simulink model "P702_NI_SoftECU"  (R2019a)
settings: Solver=ode1  StartTime=0.0  StopTime=Inf  FixedStep=0.001  RelTol=1e-3  EnableMultiTasking=on
PreLoadFcn:
  | run '.\VeriStand_BlockSet\NIVeriStandAddPaths.m'
undefined symbols (not defined in the file or in its folder): magnitude
libraries: simulink x83, simulink_extras x1
(part 60 of 76)

== system P702_NI_SoftECU/Output/Subsystem1/CAN_Signal/BCM ==
  in_port : Inport
  BCM_Lamp_Stat_0x3C3 : Subsystem
  Battery_Mgmt_24V_0x42E : Subsystem
  Battery_Mgmt_2_0x42C : Subsystem
  Battery_Mgmt_3_0x43C : Subsystem
  Battery_Mgmt_4_0x42B : Subsystem
  BodyInfo_3_0x3B3 : Subsystem
  Body_Info_10_0x3BA : Subsystem
  Body_Info_12_0x26E : Subsystem
  Body_Info_4_0x242 : Subsystem
  Body_Info_6_0x38D : Subsystem
  Body_Info_7_0x3B1 : Subsystem
  Body_Info_8_0x3B9 : Subsystem
  Body_Info_9_0x3A3 : Subsystem
  CMPS_FDM_Info_Status_0x3C7 : Subsystem
  CellPhonePassport_Stat_1_0x447 : Subsystem
  GGCC_Config_Mgmt_ID_1_0x40A : Subsystem
  GlobalClock_Data_0x84 : Subsystem
  Global_PATS_Control_Info2_0x42 : Subsystem
  Global_PATS_Control_Info_0x41 : Subsystem
  Locking_Systems_2_0x331 : Subsystem
  PaakRqData1_0x468 : Subsystem
  PaakRqData2_0x469 : Subsystem
  Personality_BCM2_Data_0x3EB : Subsystem
  Personality_BCM_Data_0x3E3 : Subsystem
  Power_Stat_0x456 : Subsystem
  RKE_Packet_0x3B6 : Subsystem
  TPM_Frame_0x3B7 : Subsystem
  Tire_Pressure_Data_0x3B5 : Subsystem
  Tire_Pressure_Data_DRW_0x3B8 : Subsystem
  Tire_Pressure_Stat_0x3B4 : Subsystem
  bus_selector : BusSelector  OutputSignals=Global_PATS_Control_Info_0x41,Global_PATS_Control_Info2_0x42,GlobalClock_Data_0x84,Body_Info_4_0x242,Body_Info_12_0x26E,Locking_Systems_2_0x331,Body_Info_6_0x38D,Body_Info_9_0x3A3,Body_Info_7_0x3B1,BodyInfo_3_0x3B3,Tire_Pressure_Stat_0x3B4,Tire_Pressure_Data_0x3B5,RKE_Packet_0x3B6,TPM_Frame_0x3B7,Tire_Pressure_Data_DRW_0x3B8,Body_Info_8_0x3B9,Body_Info_10_0x3BA,BCM_Lamp_Stat_0x3C3,CMPS_FDM_Info_Status_0x3C7,Personality_BCM_Data_0x3E3,Personality_BCM2_Data_0x3EB,GGCC_Config_Mgmt_ID_1_0x40A,Battery_Mgmt_4_0x42B,Battery_Mgmt_2_0x42C,Battery_Mgmt_24V_0x42E,Battery_Mgmt_3_0x43C,CellPhonePassport_Stat_1_0x447,Power_Stat_0x456,PaakRqData1_0x468,PaakRqData2_0x469
  wires:
  in_port/1 -> bus_selector/1  "Subsystem1"
  bus_selector/1 -> Global_PATS_Control_Info_0x41/1(in_port)  "<Global_PATS_Control_Info_0x41>"
  bus_selector/2 -> Global_PATS_Control_Info2_0x42/1(in_port)  "<Global_PATS_Control_Info2_0x42>"
  bus_selector/3 -> GlobalClock_Data_0x84/1(in_port)  "<GlobalClock_Data_0x84>"
  bus_selector/4 -> Body_Info_4_0x242/1(in_port)  "<Body_Info_4_0x242>"
  bus_selector/5 -> Body_Info_12_0x26E/1(in_port)  "<Body_Info_12_0x26E>"
  bus_selector/6 -> Locking_Systems_2_0x331/1(in_port)  "<Locking_Systems_2_0x331>"
  bus_selector/7 -> Body_Info_6_0x38D/1(in_port)  "<Body_Info_6_0x38D>"
  bus_selector/8 -> Body_Info_9_0x3A3/1(in_port)  "<Body_Info_9_0x3A3>"
  bus_selector/9 -> Body_Info_7_0x3B1/1(in_port)  "<Body_Info_7_0x3B1>"
  bus_selector/10 -> BodyInfo_3_0x3B3/1(in_port)  "<BodyInfo_3_0x3B3>"
  bus_selector/11 -> Tire_Pressure_Stat_0x3B4/1(in_port)  "<Tire_Pressure_Stat_0x3B4>"
  bus_selector/12 -> Tire_Pressure_Data_0x3B5/1(in_port)  "<Tire_Pressure_Data_0x3B5>"
  bus_selector/13 -> RKE_Packet_0x3B6/1(in_port)  "<RKE_Packet_0x3B6>"
  bus_selector/14 -> TPM_Frame_0x3B7/1(in_port)  "<TPM_Frame_0x3B7>"
  bus_selector/15 -> Tire_Pressure_Data_DRW_0x3B8/1(in_port)  "<Tire_Pressure_Data_DRW_0x3B8>"
  bus_selector/16 -> Body_Info_8_0x3B9/1(in_port)  "<Body_Info_8_0x3B9>"
  bus_selector/17 -> Body_Info_10_0x3BA/1(in_port)  "<Body_Info_10_0x3BA>"
  bus_selector/18 -> BCM_Lamp_Stat_0x3C3/1(in_port)  "<BCM_Lamp_Stat_0x3C3>"
  bus_selector/19 -> CMPS_FDM_Info_Status_0x3C7/1(in_port)  "<CMPS_FDM_Info_Status_0x3C7>"
  bus_selector/20 -> Personality_BCM_Data_0x3E3/1(in_port)  "<Personality_BCM_Data_0x3E3>"
  bus_selector/21 -> Personality_BCM2_Data_0x3EB/1(in_port)  "<Personality_BCM2_Data_0x3EB>"
  bus_selector/22 -> GGCC_Config_Mgmt_ID_1_0x40A/1(in_port)  "<GGCC_Config_Mgmt_ID_1_0x40A>"
  bus_selector/23 -> Battery_Mgmt_4_0x42B/1(in_port)  "<Battery_Mgmt_4_0x42B>"
  bus_selector/24 -> Battery_Mgmt_2_0x42C/1(in_port)  "<Battery_Mgmt_2_0x42C>"
  bus_selector/25 -> Battery_Mgmt_24V_0x42E/1(in_port)  "<Battery_Mgmt_24V_0x42E>"
  bus_selector/26 -> Battery_Mgmt_3_0x43C/1(in_port)  "<Battery_Mgmt_3_0x43C>"
  bus_selector/27 -> CellPhonePassport_Stat_1_0x447/1(in_port)  "<CellPhonePassport_Stat_1_0x447>"
  bus_selector/28 -> Power_Stat_0x456/1(in_port)  "<Power_Stat_0x456>"
  bus_selector/29 -> PaakRqData1_0x468/1(in_port)  "<PaakRqData1_0x468>"
  bus_selector/30 -> PaakRqData2_0x469/1(in_port)  "<PaakRqData2_0x469>"

== system P702_NI_SoftECU/Output/Subsystem1/CAN_Signal/DSMC ==
  in_port : Inport
  CMR_DSMC_AutoSar_NetwrkMgt : Subsystem
  DrvStatMonData : Subsystem
  TesterPhysicalResCMR_DSMC : Subsystem
  bus_selector : BusSelector  OutputSignals=CMR_DSMC_AutoSar_NetwrkMgt,DrvStatMonData,TesterPhysicalResCMR_DSMC
  wires:
  in_port/1 -> bus_selector/1  "Subsystem1"
  bus_selector/1 -> CMR_DSMC_AutoSar_NetwrkMgt/1(in_port)  "<CMR_DSMC_AutoSar_NetwrkMgt>"
  bus_selector/2 -> DrvStatMonData/1(in_port)  "<DrvStatMonData>"
  bus_selector/3 -> TesterPhysicalResCMR_DSMC/1(in_port)  "<TesterPhysicalResCMR_DSMC>"

== system P702_NI_SoftECU/Output/Subsystem1/CAN_Signal/ECM_DIESEL PCM PCM_HEV ==
  in_port : Inport
  EngBrakeData_0x165 : Subsystem
  EngVehicleSpThrottle2_0x202 : Subsystem
  EngVehicleSpThrottle_0x204 : Subsystem
  EngineClimateData_0x178 : Subsystem
  EngineData_6_0x156 : Subsystem
  EngineData_7_0x179 : Subsystem
  Engine_Clutch_Data_0x42F : Subsystem
  Gear_Shift_by_Wire_3 : Subsystem
  Global_PATS_TargetInfo_0x47 : Subsystem
  HEV_Powertrain_Data2 : Subsystem
  PCM_AutoSar_NetworkMgmt_0x595 : Subsystem
  PCM_Rapid_Data_Response_1_0x6A0 : Subsystem
  PowertrainData_10 : Subsystem
  PowertrainData_1_0x421 : Subsystem
  PowertrainData_2_0x42D : Subsystem
  PowertrainData_3_0x43E : Subsystem
  PowertrainData_6_0x205 : Subsystem
  PowertrainData_7_0x41F : Subsystem
  PowertrainData_9_0x44C : Subsystem
  Powertrain_Data_4_0x424 : Subsystem
  Powertrain_Data_5_0x43F : Subsystem
  Stop_Start_0x166 : Subsystem
  TesterPhysicalResPCM_0x7E8 : Subsystem
  TorqueDataEngFlags_0x200 : Subsystem
  TransGearData : Subsystem
  VehicleOperatingModes_0x167 : Subsystem
  bus_selector : BusSelector  OutputSignals=Global_PATS_TargetInfo_0x47,EngineData_6_0x156,EngBrakeData_0x165,Stop_Start_0x166,VehicleOperatingModes_0x167,EngineClimateData_0x178,EngineData_7_0x179,TorqueDataEngFlags_0x200,EngVehicleSpThrottle2_0x202,EngVehicleSpThrottle_0x204,PowertrainData_6_0x205,PowertrainData_7_0x41F,PowertrainData_1_0x421,Powertrain_Data_4_0x424,PowertrainData_2_0x42D,Engine_Clutch_Data_0x42F,PowertrainData_3_0x43E,Powertrain_Data_5_0x43F,PowertrainData_9_0x44C,PCM_AutoSar_NetworkMgmt_0x595,PCM_Rapid_Data_Response_1_0x6A0,TesterPhysicalResPCM_0x7E8,Gear_Shift_by_Wire_3,PowertrainData_10,TransGearData,HEV_Powertrain_Data2
  wires:
  in_port/1 -> bus_selector/1  "Subsystem1"
  bus_selector/1 -> Global_PATS_TargetInfo_0x47/1(in_port)  "<Global_PATS_TargetInfo_0x47>"
  bus_selector/2 -> EngineData_6_0x156/1(in_port)  "<EngineData_6_0x156>"
  bus_selector/3 -> EngBrakeData_0x165/1(in_port)  "<EngBrakeData_0x165>"
  bus_selector/4 -> Stop_Start_0x166/1(in_port)  "<Stop_Start_0x166>"
  bus_selector/5 -> VehicleOperatingModes_0x167/1(in_port)  "<VehicleOperatingModes_0x167>"
  bus_selector/6 -> EngineClimateData_0x178/1(in_port)  "<EngineClimateData_0x178>"
  bus_selector/7 -> EngineData_7_0x179/1(in_port)  "<EngineData_7_0x179>"
  bus_selector/8 -> TorqueDataEngFlags_0x200/1(in_port)  "<TorqueDataEngFlags_0x200>"
  bus_selector/9 -> EngVehicleSpThrottle2_0x202/1(in_port)  "<EngVehicleSpThrottle2_0x202>"
  bus_selector/10 -> EngVehicleSpThrottle_0x204/1(in_port)  "<EngVehicleSpThrottle_0x204>"
  bus_selector/11 -> PowertrainData_6_0x205/1(in_port)  "<PowertrainData_6_0x205>"
  bus_selector/12 -> PowertrainData_7_0x41F/1(in_port)  "<PowertrainData_7_0x41F>"
  bus_selector/13 -> PowertrainData_1_0x421/1(in_port)  "<PowertrainData_1_0x421>"
  bus_selector/14 -> Powertrain_Data_4_0x424/1(in_port)  "<Powertrain_Data_4_0x424>"
  bus_selector/15 -> PowertrainData_2_0x42D/1(in_port)  "<PowertrainData_2_0x42D>"
  bus_selector/16 -> Engine_Clutch_Data_0x42F/1(in_port)  "<Engine_Clutch_Data_0x42F>"
  bus_selector/17 -> PowertrainData_3_0x43E/1(in_port)  "<PowertrainData_3_0x43E>"
  bus_selector/18 -> Powertrain_Data_5_0x43F/1(in_port)  "<Powertrain_Data_5_0x43F>"
  bus_selector/19 -> PowertrainData_9_0x44C/1(in_port)  "<PowertrainData_9_0x44C>"
  bus_selector/20 -> PCM_AutoSar_NetworkMgmt_0x595/1(in_port)  "<PCM_AutoSar_NetworkMgmt_0x595>"
  bus_selector/21 -> PCM_Rapid_Data_Response_1_0x6A0/1(in_port)  "<PCM_Rapid_Data_Response_1_0x6A0>"
  bus_selector/22 -> TesterPhysicalResPCM_0x7E8/1(in_port)  "<TesterPhysicalResPCM_0x7E8>"
  bus_selector/23 -> Gear_Shift_by_Wire_3/1(in_port)  "<Gear_Shift_by_Wire_3>"
  bus_selector/24 -> PowertrainData_10/1(in_port)  "<PowertrainData_10>"
  bus_selector/25 -> TransGearData/1(in_port)  "<TransGearData>"
  bus_selector/26 -> HEV_Powertrain_Data2/1(in_port)  "<HEV_Powertrain_Data2>"

== system P702_NI_SoftECU/Output/Subsystem1/CAN_Signal/GWM ==
  in_port : Inport
  GSM : Subsystem
  Other_GWMTx : Subsystem
  RCM : Subsystem
  SCCM : Subsystem
  Tester/AutoSar : Subsystem
  bus_selector : BusSelector  OutputSignals=Other_GWMTx,RCM,SCCM,GSM,Tester/AutoSar
  wires:
  in_port/1 -> bus_selector/1  "Subsystem1"
  bus_selector/1 -> Other_GWMTx/1(in_port)  "<Other_GWMTx>"
  bus_selector/2 -> RCM/1(in_port)  "<RCM>"
  bus_selector/3 -> SCCM/1(in_port)  "<SCCM>"
  bus_selector/4 -> GSM/1(in_port)  "<GSM>"
  bus_selector/5 -> Tester/AutoSar/1(in_port)  "<Tester/AutoSar>"

== system P702_NI_SoftECU/Output/Subsystem1/CAN_Signal/PSCM ==
  in_port : Inport
  EPAS_INFO_0x82 : Subsystem
  Lane_Assist_Data3_FD1_0x3CC : Subsystem
  PSCM_AutoSar_NetwrkMgmt_0x5B5 : Subsystem
  SteeringPinion_Data_0x7E : Subsystem
  TesterPhysicalResPSCM_0x738 : Subsystem
  TrailerAid_Data2_0x417 : Subsystem
  bus_selector : BusSelector  OutputSignals=SteeringPinion_Data_0x7E,EPAS_INFO_0x82,Lane_Assist_Data3_FD1_0x3CC,TrailerAid_Data2_0x417,PSCM_AutoSar_NetwrkMgmt_0x5B5,TesterPhysicalResPSCM_0x738
  wires:
  in_port/1 -> bus_selector/1  "Subsystem1"
  bus_selector/1 -> SteeringPinion_Data_0x7E/1(in_port)  "<SteeringPinion_Data_0x7E>"
  bus_selector/2 -> EPAS_INFO_0x82/1(in_port)  "<EPAS_INFO_0x82>"
  bus_selector/3 -> Lane_Assist_Data3_FD1_0x3CC/1(in_port)  "<Lane_Assist_Data3_FD1_0x3CC>"
  bus_selector/4 -> TrailerAid_Data2_0x417/1(in_port)  "<TrailerAid_Data2_0x417>"
  bus_selector/5 -> PSCM_AutoSar_NetwrkMgmt_0x5B5/1(in_port)  "<PSCM_AutoSar_NetwrkMgmt_0x5B5>"
  bus_selector/6 -> TesterPhysicalResPSCM_0x738/1(in_port)  "<TesterPhysicalResPSCM_0x738>"

== system P702_NI_SoftECU/Output/Subsystem1/CAN_Signal/RealPCM ==
  in_port : Inport
  EngBrakeData : Subsystem
  EngVehicleSpThrottle2 : Subsystem
  bus_selector : BusSelector  OutputSignals=EngBrakeData,EngVehicleSpThrottle2,user_channel
  user_channel : Subsystem
  wires:
  in_port/1 -> bus_selector/1  "Subsystem1"
  bus_selector/1 -> EngBrakeData/1(in_port)  "<EngBrakeData>"
  bus_selector/2 -> EngVehicleSpThrottle2/1(in_port)  "<EngVehicleSpThrottle2>"
  bus_selector/3 -> user_channel/1(in_port)  "<user_channel>"

== system P702_NI_SoftECU/Output/Subsystem1/To_NI_HIL/DSMC ==
  in_port : Inport
  DrvStatMonData : Subsystem
  bus_selector : BusSelector  OutputSignals=DrvStatMonData
  wires:
  in_port/1 -> bus_selector/1  "Subsystem1"
  bus_selector/1 -> DrvStatMonData/1(in_port)  "<DrvStatMonData>"

== system P702_NI_SoftECU/Output/Subsystem1/To_NI_HIL/MRR ==
  in_port : Inport
  CAN_DET_AZIMUTH_01[rad] : Terminator
  CAN_DET_AZIMUTH_02[rad] : Terminator
  CAN_DET_AZIMUTH_03[rad] : Terminator
  CAN_DET_ELEVATION_01[rad] : Terminator
  CAN_DET_ELEVATION_02[rad] : Terminator
  CAN_DET_ELEVATION_03[rad] : Terminator
  CAN_DET_RANGE_01[m] : Terminator
  CAN_DET_RANGE_02[m] : Terminator
  CAN_DET_RANGE_03[m] : Terminator
  CAN_DET_RANGE_RATE_01[m/s] : Terminator
  CAN_DET_RANGE_RATE_02[m/s] : Terminator
  CAN_DET_RANGE_RATE_03[m/s] : Terminator
  bus_selector : BusSelector  OutputSignals=CAN_DET_RANGE_01[m],CAN_DET_RANGE_RATE_01[m/s],CAN_DET_AZIMUTH_01[rad],CAN_DET_ELEVATION_01[rad],CAN_DET_RANGE_02[m],CAN_DET_RANGE_RATE_02[m/s],CAN_DET_AZIMUTH_02[rad],CAN_DET_ELEVATION_02[rad],CAN_DET_RANGE_03[m],CAN_DET_RANGE_RATE_03[m/s],CAN_DET_AZIMUTH_03[rad],CAN_DET_ELEVATION_03[rad]
  wires:
  in_port/1 -> bus_selector/1  "Subsystem1"
  bus_selector/1 -> CAN_DET_RANGE_01[m]/1  "<CAN_DET_RANGE_01[m]>"
  bus_selector/2 -> CAN_DET_RANGE_RATE_01[m/s]/1  "<CAN_DET_RANGE_RATE_01[m/s]>"
  bus_selector/3 -> CAN_DET_AZIMUTH_01[rad]/1  "<CAN_DET_AZIMUTH_01[rad]>"
  bus_selector/4 -> CAN_DET_ELEVATION_01[rad]/1  "<CAN_DET_ELEVATION_01[rad]>"
  bus_selector/5 -> CAN_DET_RANGE_02[m]/1  "<CAN_DET_RANGE_02[m]>"
  bus_selector/6 -> CAN_DET_RANGE_RATE_02[m/s]/1  "<CAN_DET_RANGE_RATE_02[m/s]>"
  bus_selector/7 -> CAN_DET_AZIMUTH_02[rad]/1  "<CAN_DET_AZIMUTH_02[rad]>"
  bus_selector/8 -> CAN_DET_ELEVATION_02[rad]/1  "<CAN_DET_ELEVATION_02[rad]>"
  bus_selector/9 -> CAN_DET_RANGE_03[m]/1  "<CAN_DET_RANGE_03[m]>"
  bus_selector/10 -> CAN_DET_RANGE_RATE_03[m/s]/1  "<CAN_DET_RANGE_RATE_03[m/s]>"
  bus_selector/11 -> CAN_DET_AZIMUTH_03[rad]/1  "<CAN_DET_AZIMUTH_03[rad]>"
  bus_selector/12 -> CAN_DET_ELEVATION_03[rad]/1  "<CAN_DET_ELEVATION_03[rad]>"

== system P702_NI_SoftECU/Output/Subsystem1/To_NI_HIL/SRR_L ==
  in_port : Inport
  FL_SOD : Subsystem
  RL_SOD : Subsystem
  bus_selector : BusSelector  OutputSignals=RL_SOD,FL_SOD
  wires:
  in_port/1 -> bus_selector/1  "Subsystem1"
  bus_selector/1 -> RL_SOD/1(in_port)  "<RL_SOD>"
  bus_selector/2 -> FL_SOD/1(in_port)  "<FL_SOD>"

== system P702_NI_SoftECU/Output/Subsystem1/To_NI_HIL/SRR_R ==
  in_port : Inport
  FR_SOD : Subsystem
  RR_SOD : Subsystem
  bus_selector : BusSelector  OutputSignals=RR_SOD,FR_SOD
  wires:
  in_port/1 -> bus_selector/1  "Subsystem1"
  bus_selector/1 -> RR_SOD/1(in_port)  "<RR_SOD>"
  bus_selector/2 -> FR_SOD/1(in_port)  "<FR_SOD>"

== system P702_NI_SoftECU/Output/Subsystem1/To_NI_HIL/Soft_ABS ==
  in_port : Inport
  ABS_BrkBst_Data : Subsystem
  Accel_Data : Subsystem
  BrakeSnData_3 : Subsystem
  BrakeSnData_4 : Subsystem
  BrakeSnData_5 : Subsystem
  BrakeSysFeatures : Subsystem
  BrakeSysFeatures_2 : Subsystem
  DesiredTorqBrk : Subsystem
  ToCarSim : Subsystem
  WheelData : Subsystem
  WheelSpeed : Subsystem
  Yaw_Data : Subsystem
  bus_selector : BusSelector  OutputSignals=WheelSpeed,WheelData,Accel_Data,Yaw_Data,BrakeSnData_3,DesiredTorqBrk,BrakeSnData_4,BrakeSysFeatures,BrakeSnData_5,ToCarSim,ABS_BrkBst_Data,BrakeSysFeatures_2
  wires:
  in_port/1 -> bus_selector/1  "Subsystem1"
  bus_selector/1 -> WheelSpeed/1(in_port)  "<WheelSpeed>"
  bus_selector/2 -> WheelData/1(in_port)  "<WheelData>"
  bus_selector/3 -> Accel_Data/1(in_port)  "<Accel_Data>"
  bus_selector/4 -> Yaw_Data/1(in_port)  "<Yaw_Data>"
  bus_selector/5 -> BrakeSnData_3/1(in_port)  "<BrakeSnData_3>"
  bus_selector/6 -> DesiredTorqBrk/1(in_port)  "<DesiredTorqBrk>"
  bus_selector/7 -> BrakeSnData_4/1(in_port)  "<BrakeSnData_4>"
  bus_selector/8 -> BrakeSysFeatures/1(in_port)  "<BrakeSysFeatures>"
  bus_selector/9 -> BrakeSnData_5/1(in_port)  "<BrakeSnData_5>"
  bus_selector/10 -> ToCarSim/1(in_port)  "<ToCarSim>"
  bus_selector/11 -> ABS_BrkBst_Data/1(in_port)  "<ABS_BrkBst_Data>"
  bus_selector/12 -> BrakeSysFeatures_2/1(in_port)  "<BrakeSysFeatures_2>"

== system P702_NI_SoftECU/Output/Subsystem1/To_NI_HIL/Soft_BCM ==
  in_port : Inport
  BodyInfo_3 : Subsystem
  Cluster_Info1 : Subsystem
  GGCC_Config_Mgmt_ID : Subsystem
  Personality_BCM2_Data : Subsystem
  bus_selector : BusSelector  OutputSignals=signal1,Cluster_Info1,BodyInfo_3,GGCC_Config_Mgmt_ID,signal5,signal6,Personality_BCM2_Data
  signal1 : Terminator
  signal5 : Terminator
  signal6 : Terminator
  wires:
  in_port/1 -> bus_selector/1  "Subsystem1"
  bus_selector/1 -> signal1/1  "<signal1>"
  bus_selector/5 -> signal5/1  "<signal5>"
  bus_selector/6 -> signal6/1  "<signal6>"
  bus_selector/2 -> Cluster_Info1/1(in_port)  "<Cluster_Info1>"
  bus_selector/3 -> BodyInfo_3/1(in_port)  "<BodyInfo_3>"
  bus_selector/4 -> GGCC_Config_Mgmt_ID/1(in_port)  "<GGCC_Config_Mgmt_ID>"
  bus_selector/7 -> Personality_BCM2_Data/1(in_port)  "<Personality_BCM2_Data>"

== system P702_NI_SoftECU/Output/Subsystem1/To_NI_HIL/Soft_ECM ==
  in_port : Inport
  EngBrakeData : Subsystem
  EngVehicleSpThrottle : Subsystem
  EngVehicleSpThrottle2 : Subsystem
  bus_selector : BusSelector  OutputSignals=EngVehicleSpThrottle2,EngBrakeData,EngVehicleSpThrottle
  wires:
  in_port/1 -> bus_selector/1  "Subsystem1"
  bus_selector/1 -> EngVehicleSpThrottle2/1(in_port)  "<EngVehicleSpThrottle2>"
  bus_selector/2 -> EngBrakeData/1(in_port)  "<EngBrakeData>"
  bus_selector/3 -> EngVehicleSpThrottle/1(in_port)  "<EngVehicleSpThrottle>"

== system P702_NI_SoftECU/Output/Subsystem1/To_NI_HIL/Soft_MRR ==
  in_port : Inport
  MRR_Detection : Subsystem
  NumOfDetections : Terminator
  bus_selector : BusSelector  OutputSignals=MRR_Detection,NumOfDetections
  wires:
  in_port/1 -> bus_selector/1  "Subsystem1"
  bus_selector/2 -> NumOfDetections/1  "<NumOfDetections>"
  bus_selector/1 -> MRR_Detection/1(in_port)  "<MRR_Detection>"

== system P702_NI_SoftECU/Output/Subsystem1/To_NI_HIL/Soft_PCM ==
  in_port : Inport
  EngBrakeData : Subsystem
  EngVehicleSpThottle2 : Subsystem
  EngVehicleSpThrottle : Subsystem
  EngineClimateData : Subsystem
  EngineClutchData : Subsystem
  EngineData_7 : Subsystem
  PowertrainData_10 : Subsystem
  TorqueDataEngFlags : Subsystem
  VehicleOperatingModes : Subsystem
  bus_selector : BusSelector  OutputSignals=EngBrakeData,EngineClimateData,EngineClutchData,EngVehicleSpThrottle,EngVehicleSpThottle2,VehicleOperatingModes,EngineData_7,TorqueDataEngFlags,PowertrainData_10
  wires:
  in_port/1 -> bus_selector/1  "Subsystem1"
  bus_selector/1 -> EngBrakeData/1(in_port)  "<EngBrakeData>"
  bus_selector/2 -> EngineClimateData/1(in_port)  "<EngineClimateData>"
  bus_selector/3 -> EngineClutchData/1(in_port)  "<EngineClutchData>"
  bus_selector/4 -> EngVehicleSpThrottle/1(in_port)  "<EngVehicleSpThrottle>"
  bus_selector/5 -> EngVehicleSpThottle2/1(in_port)  "<EngVehicleSpThottle2>"
  bus_selector/6 -> VehicleOperatingModes/1(in_port)  "<VehicleOperatingModes>"
  bus_selector/7 -> EngineData_7/1(in_port)  "<EngineData_7>"
  bus_selector/8 -> TorqueDataEngFlags/1(in_port)  "<TorqueDataEngFlags>"
  bus_selector/9 -> PowertrainData_10/1(in_port)  "<PowertrainData_10>"

== system P702_NI_SoftECU/Output/Subsystem1/To_NI_HIL/Soft_PSCM ==
  in_port : Inport
  Angle_SteeringWheel : Terminator
  StePinCompAnEst_D_Qf : Terminator
  StePinRelInit_An_Sns : Terminator
  StePw_B_Rq : Terminator
  SteWhlAngCounter : Terminator
  WhlAngleCs : Terminator
  bus_selector : BusSelector  OutputSignals=Angle_SteeringWheel,SteWhlAngCounter,WhlAngleCs,StePinRelInit_An_Sns,StePw_B_Rq,StePinCompAnEst_D_Qf
  wires:
  in_port/1 -> bus_selector/1  "Subsystem1"
  bus_selector/1 -> Angle_SteeringWheel/1  "<Angle_SteeringWheel>"
  bus_selector/2 -> SteWhlAngCounter/1  "<SteWhlAngCounter>"
  bus_selector/3 -> WhlAngleCs/1  "<WhlAngleCs>"
  bus_selector/4 -> StePinRelInit_An_Sns/1  "<StePinRelInit_An_Sns>"
  bus_selector/5 -> StePw_B_Rq/1  "<StePw_B_Rq>"
  bus_selector/6 -> StePinCompAnEst_D_Qf/1  "<StePinCompAnEst_D_Qf>"

== system P702_NI_SoftECU/Output/Subsystem1/To_NI_HIL/Soft_RCM ==
  in_port : Inport
  Accel_Data : Subsystem
  RCMStatusMessage2 : Subsystem
  Yaw_Data : Subsystem
  bus_selector : BusSelector  OutputSignals=Accel_Data,Yaw_Data,RCMStatusMessage2
  wires:
  in_port/1 -> bus_selector/1  "Subsystem1"
  bus_selector/1 -> Accel_Data/1(in_port)  "<Accel_Data>"
  bus_selector/2 -> Yaw_Data/1(in_port)  "<Yaw_Data>"
  bus_selector/3 -> RCMStatusMessage2/1(in_port)  "<RCMStatusMessage2>"

== system P702_NI_SoftECU/Output/Subsystem1/To_NI_HIL/Soft_SCCM ==
  in_port : Inport
  Steering_Data : Subsystem
  Steering_Wheel_Data2 : Subsystem
  bus_selector : BusSelector  OutputSignals=Steering_Data,Steering_Wheel_Data2
  wires:
  in_port/1 -> bus_selector/1  "Subsystem1"
  bus_selector/1 -> Steering_Data/1(in_port)  "<Steering_Data>"
  bus_selector/2 -> Steering_Wheel_Data2/1(in_port)  "<Steering_Wheel_Data2>"

== system P702_NI_SoftECU/Output/Subsystem1/To_NI_HIL/Soft_TCM ==
  in_port : Inport
  TransGearData : Subsystem
  bus_selector : BusSelector  OutputSignals=TransGearData
  wires:
  in_port/1 -> bus_selector/1  "Subsystem1"
  bus_selector/1 -> TransGearData/1(in_port)  "<TransGearData>"

== system P702_NI_SoftECU/Output/Subsystem2/CAN_Signal/ABS_ESC ==
  ABS_AutoSar_NetworkMgt_0x596 : Subsystem
  ABS_BrkBst_Data_0x4B0 : Subsystem
  ABS_Rapid_Data_Response_1_0x6B0 : Subsystem
  ABS_Rapid_Data_Response_2_0x6B1 : Subsystem
  ActiveFronSteering_Req_0x88 : Subsystem
  BrakeSnData_3_0x77 : Subsystem
  BrakeSnData_4_0x7D : Subsystem
  BrakeSnData_5_0x76 : Subsystem
  BrakeSnData_6_0x414 : Subsystem
  BrakeSysFeatures_0x415 : Subsystem
  BrakeSysFeatures_2_0x416 : Subsystem
  BrakeSysFeatures_3_0x41E : Subsystem
  DesiredTorqBrk_0x213 : Subsystem
  DesiredTorqBrk_2_0x214 : Subsystem
  Global_PATS_SubTarget_0x49 : Subsystem
  SelectDriveModeData2_0x44E : Subsystem
  SelectDriveModeData_0x420 : Subsystem
  SteeringPinion_Data2_0x7F : Subsystem
  TesterPhysicalResABS_0x768 : Subsystem
  TrailerBrakeData_0x412 : Subsystem
  WheelData_0x216 : Subsystem
  WheelSpeed_0x217 : Subsystem
  bus_creator : BusCreator  Inputs=22
  out_port : Outport
  wires:
  bus_creator/1 -> out_port/1  "Subsystem2"
  Global_PATS_SubTarget_0x49/1(out_port) -> bus_creator/1  "Global_PATS_SubTarget_0x49"
  BrakeSnData_5_0x76/1(out_port) -> bus_creator/2  "BrakeSnData_5_0x76"
  BrakeSnData_3_0x77/1(out_port) -> bus_creator/3  "BrakeSnData_3_0x77"
  BrakeSnData_4_0x7D/1(out_port) -> bus_creator/4  "BrakeSnData_4_0x7D"
  SteeringPinion_Data2_0x7F/1(out_port) -> bus_creator/5  "SteeringPinion_Data2_0x7F"
  ActiveFronSteering_Req_0x88/1(out_port) -> bus_creator/6  "ActiveFronSteering_Req_0x88"
  DesiredTorqBrk_0x213/1(out_port) -> bus_creator/7  "DesiredTorqBrk_0x213"
  DesiredTorqBrk_2_0x214/1(out_port) -> bus_creator/8  "DesiredTorqBrk_2_0x214"
  WheelData_0x216/1(out_port) -> bus_creator/9  "WheelData_0x216"
  WheelSpeed_0x217/1(out_port) -> bus_creator/10  "WheelSpeed_0x217"
  TrailerBrakeData_0x412/1(out_port) -> bus_creator/11  "TrailerBrakeData_0x412"
  BrakeSnData_6_0x414/1(out_port) -> bus_creator/12  "BrakeSnData_6_0x414"
  BrakeSysFeatures_0x415/1(out_port) -> bus_creator/13  "BrakeSysFeatures_0x415"
  BrakeSysFeatures_2_0x416/1(out_port) -> bus_creator/14  "BrakeSysFeatures_2_0x416"
  BrakeSysFeatures_3_0x41E/1(out_port) -> bus_creator/15  "BrakeSysFeatures_3_0x41E"
  SelectDriveModeData_0x420/1(out_port) -> bus_creator/16  "SelectDriveModeData_0x420"
  SelectDriveModeData2_0x44E/1(out_port) -> bus_creator/17  "SelectDriveModeData2_0x44E"
  ABS_BrkBst_Data_0x4B0/1(out_port) -> bus_creator/18  "ABS_BrkBst_Data_0x4B0"
  ABS_AutoSar_NetworkMgt_0x596/1(out_port) -> bus_creator/19  "ABS_AutoSar_NetworkMgt_0x596"
  ABS_Rapid_Data_Response_1_0x6B0/1(out_port) -> bus_creator/20  "ABS_Rapid_Data_Response_1_0x6B0"
  ABS_Rapid_Data_Response_2_0x6B1/1(out_port) -> bus_creator/21  "ABS_Rapid_Data_Response_2_0x6B1"
  TesterPhysicalResABS_0x768/1(out_port) -> bus_creator/22  "TesterPhysicalResABS_0x768"

== system P702_NI_SoftECU/Output/Subsystem2/CAN_Signal/ADAS ==
  ACCDATA : Subsystem
  ACCDATA_2 : Subsystem
  bus_creator : BusCreator  Inputs=2
  out_port : Outport
  wires:
  bus_creator/1 -> out_port/1  "Subsystem2"
  ACCDATA/1(out_port) -> bus_creator/1  "ACCDATA"
  ACCDATA_2/1(out_port) -> bus_creator/2  "ACCDATA_2"

== system P702_NI_SoftECU/Output/Subsystem2/CAN_Signal/BCM ==
  BCM_Lamp_Stat_0x3C3 : Subsystem
  Battery_Mgmt_24V_0x42E : Subsystem
  Battery_Mgmt_2_0x42C : Subsystem
  Battery_Mgmt_3_0x43C : Subsystem
  Battery_Mgmt_4_0x42B : Subsystem
  BodyInfo_3_0x3B3 : Subsystem
  Body_Info_10_0x3BA : Subsystem
  Body_Info_12_0x26E : Subsystem
  Body_Info_4_0x242 : Subsystem
  Body_Info_6_0x38D : Subsystem
  Body_Info_7_0x3B1 : Subsystem
  Body_Info_8_0x3B9 : Subsystem
  Body_Info_9_0x3A3 : Subsystem
  CMPS_FDM_Info_Status_0x3C7 : Subsystem
  CellPhonePassport_Stat_1_0x447 : Subsystem
  GGCC_Config_Mgmt_ID_1_0x40A : Subsystem
  GlobalClock_Data_0x84 : Subsystem
  Global_PATS_Control_Info2_0x42 : Subsystem
  Global_PATS_Control_Info_0x41 : Subsystem
  Locking_Systems_2_0x331 : Subsystem
  PaakRqData1_0x468 : Subsystem
  PaakRqData2_0x469 : Subsystem
  Personality_BCM2_Data_0x3EB : Subsystem
  Personality_BCM_Data_0x3E3 : Subsystem
  Power_Stat_0x456 : Subsystem
  RKE_Packet_0x3B6 : Subsystem
  TPM_Frame_0x3B7 : Subsystem
  Tire_Pressure_Data_0x3B5 : Subsystem
  Tire_Pressure_Data_DRW_0x3B8 : Subsystem
  Tire_Pressure_Stat_0x3B4 : Subsystem
  bus_creator : BusCreator  Inputs=30
  out_port : Outport
  wires:
  bus_creator/1 -> out_port/1  "Subsystem2"
  Global_PATS_Control_Info_0x41/1(out_port) -> bus_creator/1  "Global_PATS_Control_Info_0x41"
  Global_PATS_Control_Info2_0x42/1(out_port) -> bus_creator/2  "Global_PATS_Control_Info2_0x42"
  GlobalClock_Data_0x84/1(out_port) -> bus_creator/3  "GlobalClock_Data_0x84"
  Body_Info_4_0x242/1(out_port) -> bus_creator/4  "Body_Info_4_0x242"
  Body_Info_12_0x26E/1(out_port) -> bus_creator/5  "Body_Info_12_0x26E"
  Locking_Systems_2_0x331/1(out_port) -> bus_creator/6  "Locking_Systems_2_0x331"
  Body_Info_6_0x38D/1(out_port) -> bus_creator/7  "Body_Info_6_0x38D"
  Body_Info_9_0x3A3/1(out_port) -> bus_creator/8  "Body_Info_9_0x3A3"
  Body_Info_7_0x3B1/1(out_port) -> bus_creator/9  "Body_Info_7_0x3B1"
  BodyInfo_3_0x3B3/1(out_port) -> bus_creator/10  "BodyInfo_3_0x3B3"
  Tire_Pressure_Stat_0x3B4/1(out_port) -> bus_creator/11  "Tire_Pressure_Stat_0x3B4"
  Tire_Pressure_Data_0x3B5/1(out_port) -> bus_creator/12  "Tire_Pressure_Data_0x3B5"
  RKE_Packet_0x3B6/1(out_port) -> bus_creator/13  "RKE_Packet_0x3B6"
  TPM_Frame_0x3B7/1(out_port) -> bus_creator/14  "TPM_Frame_0x3B7"
  Tire_Pressure_Data_DRW_0x3B8/1(out_port) -> bus_creator/15  "Tire_Pressure_Data_DRW_0x3B8"
  Body_Info_8_0x3B9/1(out_port) -> bus_creator/16  "Body_Info_8_0x3B9"
  Body_Info_10_0x3BA/1(out_port) -> bus_creator/17  "Body_Info_10_0x3BA"
  BCM_Lamp_Stat_0x3C3/1(out_port) -> bus_creator/18  "BCM_Lamp_Stat_0x3C3"
  CMPS_FDM_Info_Status_0x3C7/1(out_port) -> bus_creator/19  "CMPS_FDM_Info_Status_0x3C7"
  Personality_BCM_Data_0x3E3/1(out_port) -> bus_creator/20  "Personality_BCM_Data_0x3E3"
  Personality_BCM2_Data_0x3EB/1(out_port) -> bus_creator/21  "Personality_BCM2_Data_0x3EB"
  GGCC_Config_Mgmt_ID_1_0x40A/1(out_port) -> bus_creator/22  "GGCC_Config_Mgmt_ID_1_0x40A"
  Battery_Mgmt_4_0x42B/1(out_port) -> bus_creator/23  "Battery_Mgmt_4_0x42B"
  Battery_Mgmt_2_0x42C/1(out_port) -> bus_creator/24  "Battery_Mgmt_2_0x42C"
  Battery_Mgmt_24V_0x42E/1(out_port) -> bus_creator/25  "Battery_Mgmt_24V_0x42E"
  Battery_Mgmt_3_0x43C/1(out_port) -> bus_creator/26  "Battery_Mgmt_3_0x43C"
  CellPhonePassport_Stat_1_0x447/1(out_port) -> bus_creator/27  "CellPhonePassport_Stat_1_0x447"
  Power_Stat_0x456/1(out_port) -> bus_creator/28  "Power_Stat_0x456"
  PaakRqData1_0x468/1(out_port) -> bus_creator/29  "PaakRqData1_0x468"
  PaakRqData2_0x469/1(out_port) -> bus_creator/30  "PaakRqData2_0x469"

== system P702_NI_SoftECU/Output/Subsystem2/CAN_Signal/DSMC ==
  CMR_DSMC_AutoSar_NetwrkMgt : Subsystem
  DrvStatMonData : Subsystem
  TesterPhysicalResCMR_DSMC : Subsystem
  bus_creator : BusCreator  Inputs=3
  out_port : Outport
  wires:
  bus_creator/1 -> out_port/1  "Subsystem2"
  CMR_DSMC_AutoSar_NetwrkMgt/1(out_port) -> bus_creator/1  "CMR_DSMC_AutoSar_NetwrkMgt"
  DrvStatMonData/1(out_port) -> bus_creator/2  "DrvStatMonData"
  TesterPhysicalResCMR_DSMC/1(out_port) -> bus_creator/3  "TesterPhysicalResCMR_DSMC"

== system P702_NI_SoftECU/Output/Subsystem2/CAN_Signal/ECM_DIESEL PCM PCM_HEV ==
  EngBrakeData_0x165 : Subsystem
  EngVehicleSpThrottle2_0x202 : Subsystem
  EngVehicleSpThrottle_0x204 : Subsystem
  EngineClimateData_0x178 : Subsystem
  EngineData_6_0x156 : Subsystem
  EngineData_7_0x179 : Subsystem
  Engine_Clutch_Data_0x42F : Subsystem
  Gear_Shift_by_Wire_3 : Subsystem
  Global_PATS_TargetInfo_0x47 : Subsystem
  HEV_Powertrain_Data2 : Subsystem
  PCM_AutoSar_NetworkMgmt_0x595 : Subsystem
  PCM_Rapid_Data_Response_1_0x6A0 : Subsystem
  PowertrainData_10 : Subsystem
  PowertrainData_1_0x421 : Subsystem
  PowertrainData_2_0x42D : Subsystem
  PowertrainData_3_0x43E : Subsystem
  PowertrainData_6_0x205 : Subsystem
  PowertrainData_7_0x41F : Subsystem
  PowertrainData_9_0x44C : Subsystem
  Powertrain_Data_4_0x424 : Subsystem
  Powertrain_Data_5_0x43F : Subsystem
  Stop_Start_0x166 : Subsystem
  TesterPhysicalResPCM_0x7E8 : Subsystem
  TorqueDataEngFlags_0x200 : Subsystem
  TransGearData : Subsystem
  VehicleOperatingModes_0x167 : Subsystem
  bus_creator : BusCreator  Inputs=26
  out_port : Outport
  wires:
  bus_creator/1 -> out_port/1  "Subsystem2"
  Global_PATS_TargetInfo_0x47/1(out_port) -> bus_creator/1  "Global_PATS_TargetInfo_0x47"
  EngineData_6_0x156/1(out_port) -> bus_creator/2  "EngineData_6_0x156"
  EngBrakeData_0x165/1(out_port) -> bus_creator/3  "EngBrakeData_0x165"
  Stop_Start_0x166/1(out_port) -> bus_creator/4  "Stop_Start_0x166"
  VehicleOperatingModes_0x167/1(out_port) -> bus_creator/5  "VehicleOperatingModes_0x167"
  EngineClimateData_0x178/1(out_port) -> bus_creator/6  "EngineClimateData_0x178"
  EngineData_7_0x179/1(out_port) -> bus_creator/7  "EngineData_7_0x179"
  TorqueDataEngFlags_0x200/1(out_port) -> bus_creator/8  "TorqueDataEngFlags_0x200"
  EngVehicleSpThrottle2_0x202/1(out_port) -> bus_creator/9  "EngVehicleSpThrottle2_0x202"
  EngVehicleSpThrottle_0x204/1(out_port) -> bus_creator/10  "EngVehicleSpThrottle_0x204"
  PowertrainData_6_0x205/1(out_port) -> bus_creator/11  "PowertrainData_6_0x205"
  PowertrainData_7_0x41F/1(out_port) -> bus_creator/12  "PowertrainData_7_0x41F"
  PowertrainData_1_0x421/1(out_port) -> bus_creator/13  "PowertrainData_1_0x421"
  Powertrain_Data_4_0x424/1(out_port) -> bus_creator/14  "Powertrain_Data_4_0x424"
  PowertrainData_2_0x42D/1(out_port) -> bus_creator/15  "PowertrainData_2_0x42D"
  Engine_Clutch_Data_0x42F/1(out_port) -> bus_creator/16  "Engine_Clutch_Data_0x42F"
  PowertrainData_3_0x43E/1(out_port) -> bus_creator/17  "PowertrainData_3_0x43E"
  Powertrain_Data_5_0x43F/1(out_port) -> bus_creator/18  "Powertrain_Data_5_0x43F"
  PowertrainData_9_0x44C/1(out_port) -> bus_creator/19  "PowertrainData_9_0x44C"
  PCM_AutoSar_NetworkMgmt_0x595/1(out_port) -> bus_creator/20  "PCM_AutoSar_NetworkMgmt_0x595"
  PCM_Rapid_Data_Response_1_0x6A0/1(out_port) -> bus_creator/21  "PCM_Rapid_Data_Response_1_0x6A0"
  TesterPhysicalResPCM_0x7E8/1(out_port) -> bus_creator/22  "TesterPhysicalResPCM_0x7E8"
  Gear_Shift_by_Wire_3/1(out_port) -> bus_creator/23  "Gear_Shift_by_Wire_3"
  PowertrainData_10/1(out_port) -> bus_creator/24  "PowertrainData_10"
  TransGearData/1(out_port) -> bus_creator/25  "TransGearData"
  HEV_Powertrain_Data2/1(out_port) -> bus_creator/26  "HEV_Powertrain_Data2"

== system P702_NI_SoftECU/Output/Subsystem2/CAN_Signal/GWM ==
  in : Inport
  GSM : Subsystem
  Other_GWMTx : Subsystem
  RCM : Subsystem
  SCCM : Subsystem
  Tester/AutoSar : Subsystem
  bus_creator : BusCreator  Inputs=5
  bus_selector : BusSelector  OutputSignals=Other_GWMTx,RCM,SCCM,GSM,Tester/AutoSar
  out_port : Outport
  wires:
  bus_creator/1 -> out_port/1  "Subsystem2"
  Other_GWMTx/1(out_port) -> bus_creator/1  "Other_GWMTx"
  RCM/1(out_port) -> bus_creator/2  "RCM"
  SCCM/1(out_port) -> bus_creator/3  "SCCM"
  GSM/1(out_port) -> bus_creator/4  "GSM"
  Tester/AutoSar/1(out_port) -> bus_creator/5  "Tester//AutoSar"
  bus_selector/1 -> Other_GWMTx/1(in)  "<Other_GWMTx>"
  bus_selector/2 -> RCM/1(in)  "<RCM>"
  bus_selector/3 -> SCCM/1(in)  "<SCCM>"
  bus_selector/4 -> GSM/1(in)  "<GSM>"
  bus_selector/5 -> Tester/AutoSar/1(in)  "<Tester/AutoSar>"
  in/1 -> bus_selector/1

== system P702_NI_SoftECU/Output/Subsystem2/CAN_Signal/PSCM ==
  EPAS_INFO_0x82 : Subsystem
  Lane_Assist_Data3_FD1_0x3CC : Subsystem
  PSCM_AutoSar_NetwrkMgmt_0x5B5 : Subsystem
  SteeringPinion_Data_0x7E : Subsystem
  TesterPhysicalResPSCM_0x738 : Subsystem
  TrailerAid_Data2_0x417 : Subsystem
  bus_creator : BusCreator  Inputs=6
  out_port : Outport
  wires:
  bus_creator/1 -> out_port/1  "Subsystem2"
  SteeringPinion_Data_0x7E/1(out_port) -> bus_creator/1  "SteeringPinion_Data_0x7E"
  EPAS_INFO_0x82/1(out_port) -> bus_creator/2  "EPAS_INFO_0x82"
  Lane_Assist_Data3_FD1_0x3CC/1(out_port) -> bus_creator/3  "Lane_Assist_Data3_FD1_0x3CC"
  TrailerAid_Data2_0x417/1(out_port) -> bus_creator/4  "TrailerAid_Data2_0x417"
  PSCM_AutoSar_NetwrkMgmt_0x5B5/1(out_port) -> bus_creator/5  "PSCM_AutoSar_NetwrkMgmt_0x5B5"
  TesterPhysicalResPSCM_0x738/1(out_port) -> bus_creator/6  "TesterPhysicalResPSCM_0x738"

== system P702_NI_SoftECU/Output/Subsystem2/CAN_Signal/RealPCM ==
  EngBrakeData : Subsystem
  EngVehicleSpThrottle2 : Subsystem
  bus_creator : BusCreator  Inputs=3
  user_channel : Subsystem
  out_port : Outport
  wires:
  bus_creator/1 -> out_port/1  "Subsystem2"
  EngBrakeData/1(out_port) -> bus_creator/1  "EngBrakeData"
  EngVehicleSpThrottle2/1(out_port) -> bus_creator/2  "EngVehicleSpThrottle2"
  user_channel/1(out_port) -> bus_creator/3  "user_channel"

== system P702_NI_SoftECU/Output/Subsystem2/To_NI_HIL/DSMC ==
  DrvStatMonData : Subsystem
  bus_creator : BusCreator  Inputs=1
  out_port : Outport
  wires:
  bus_creator/1 -> out_port/1  "Subsystem2"
  DrvStatMonData/1(out_port) -> bus_creator/1  "DrvStatMonData"

== system P702_NI_SoftECU/Output/Subsystem2/To_NI_HIL/MRR ==
  CAN_DET_AZIMUTH_01[rad] : Constant  Value=0
  CAN_DET_AZIMUTH_02[rad] : Constant  Value=0
  CAN_DET_AZIMUTH_03[rad] : Constant  Value=0
  CAN_DET_ELEVATION_01[rad] : Constant  Value=0
  CAN_DET_ELEVATION_02[rad] : Constant  Value=0
  CAN_DET_ELEVATION_03[rad] : Constant  Value=0
  CAN_DET_RANGE_01[m] : Constant  Value=0
  CAN_DET_RANGE_02[m] : Constant  Value=0
  CAN_DET_RANGE_03[m] : Constant  Value=0
  CAN_DET_RANGE_RATE_01[m/s] : Constant
  CAN_DET_RANGE_RATE_02[m/s] : Constant
  CAN_DET_RANGE_RATE_03[m/s] : Constant
  bus_creator : BusCreator  Inputs=12
  out_port : Outport
  wires:
  bus_creator/1 -> out_port/1  "Subsystem2"
  CAN_DET_RANGE_01[m]/1 -> bus_creator/1  "CAN_DET_RANGE_01[m]"
  CAN_DET_RANGE_RATE_01[m/s]/1 -> bus_creator/2  "CAN_DET_RANGE_RATE_01[m//s]"
  CAN_DET_AZIMUTH_01[rad]/1 -> bus_creator/3  "CAN_DET_AZIMUTH_01[rad]"
  CAN_DET_ELEVATION_01[rad]/1 -> bus_creator/4  "CAN_DET_ELEVATION_01[rad]"
  CAN_DET_RANGE_02[m]/1 -> bus_creator/5  "CAN_DET_RANGE_02[m]"
  CAN_DET_RANGE_RATE_02[m/s]/1 -> bus_creator/6  "CAN_DET_RANGE_RATE_02[m//s]"
  CAN_DET_AZIMUTH_02[rad]/1 -> bus_creator/7  "CAN_DET_AZIMUTH_02[rad]"
  CAN_DET_ELEVATION_02[rad]/1 -> bus_creator/8  "CAN_DET_ELEVATION_02[rad]"
  CAN_DET_RANGE_03[m]/1 -> bus_creator/9  "CAN_DET_RANGE_03[m]"
  CAN_DET_RANGE_RATE_03[m/s]/1 -> bus_creator/10  "CAN_DET_RANGE_RATE_03[m//s]"
  CAN_DET_AZIMUTH_03[rad]/1 -> bus_creator/11  "CAN_DET_AZIMUTH_03[rad]"
  CAN_DET_ELEVATION_03[rad]/1 -> bus_creator/12  "CAN_DET_ELEVATION_03[rad]"

== system P702_NI_SoftECU/Output/Subsystem2/To_NI_HIL/SRR_L ==
  FL_SOD : Subsystem
  RL_SOD : Subsystem
  bus_creator : BusCreator  Inputs=2
  out_port : Outport
  wires:
  bus_creator/1 -> out_port/1  "Subsystem2"
  RL_SOD/1(out_port) -> bus_creator/1  "RL_SOD"
  FL_SOD/1(out_port) -> bus_creator/2  "FL_SOD"

== system P702_NI_SoftECU/Output/Subsystem2/To_NI_HIL/SRR_R ==
  FR_SOD : Subsystem
  RR_SOD : Subsystem
  bus_creator : BusCreator  Inputs=2
  out_port : Outport
  wires:
  bus_creator/1 -> out_port/1  "Subsystem2"
  RR_SOD/1(out_port) -> bus_creator/1  "RR_SOD"
  FR_SOD/1(out_port) -> bus_creator/2  "FR_SOD"

== system P702_NI_SoftECU/Output/Subsystem2/To_NI_HIL/Soft_ABS ==
  ABS_BrkBst_Data : Subsystem
  Accel_Data : Subsystem
  BrakeSnData_3 : Subsystem
  BrakeSnData_4 : Subsystem
  BrakeSnData_5 : Subsystem
  BrakeSysFeatures : Subsystem
  BrakeSysFeatures_2 : Subsystem
  DesiredTorqBrk : Subsystem
  ToCarSim : Subsystem
  WheelData : Subsystem
  WheelSpeed : Subsystem
  Yaw_Data : Subsystem
  bus_creator : BusCreator  Inputs=12
  out_port : Outport
  wires:
  bus_creator/1 -> out_port/1  "Subsystem2"
  WheelSpeed/1(out_port) -> bus_creator/1  "WheelSpeed"
  WheelData/1(out_port) -> bus_creator/2  "WheelData"
  Accel_Data/1(out_port) -> bus_creator/3  "Accel_Data"
  Yaw_Data/1(out_port) -> bus_creator/4  "Yaw_Data"
  BrakeSnData_3/1(out_port) -> bus_creator/5  "BrakeSnData_3"
  DesiredTorqBrk/1(out_port) -> bus_creator/6  "DesiredTorqBrk"
  BrakeSnData_4/1(out_port) -> bus_creator/7  "BrakeSnData_4"
  BrakeSysFeatures/1(out_port) -> bus_creator/8  "BrakeSysFeatures"
  BrakeSnData_5/1(out_port) -> bus_creator/9  "BrakeSnData_5"
  ToCarSim/1(out_port) -> bus_creator/10  "ToCarSim"
  ABS_BrkBst_Data/1(out_port) -> bus_creator/11  "ABS_BrkBst_Data"
  BrakeSysFeatures_2/1(out_port) -> bus_creator/12  "BrakeSysFeatures_2"

== system P702_NI_SoftECU/Output/Subsystem2/To_NI_HIL/Soft_BCM ==
  BodyInfo_3 : Subsystem
  Cluster_Info1 : Subsystem
  GGCC_Config_Mgmt_ID : Subsystem
  Personality_BCM2_Data : Subsystem
  bus_creator : BusCreator  Inputs=7
  signal1 : Constant  Value=0
  signal5 : Constant  Value=0
  signal6 : Constant  Value=0
  out_port : Outport
  wires:
  bus_creator/1 -> out_port/1  "Subsystem2"
  signal1/1 -> bus_creator/1  "signal1"
  signal5/1 -> bus_creator/5  "signal5"
  signal6/1 -> bus_creator/6  "signal6"
  Cluster_Info1/1(out_port) -> bus_creator/2  "Cluster_Info1"
  BodyInfo_3/1(out_port) -> bus_creator/3  "BodyInfo_3"
  GGCC_Config_Mgmt_ID/1(out_port) -> bus_creator/4  "GGCC_Config_Mgmt_ID"
  Personality_BCM2_Data/1(out_port) -> bus_creator/7  "Personality_BCM2_Data"

== system P702_NI_SoftECU/Output/Subsystem2/To_NI_HIL/Soft_ECM ==
  EngBrakeData : Subsystem
  EngVehicleSpThrottle : Subsystem
  EngVehicleSpThrottle2 : Subsystem
  bus_creator : BusCreator  Inputs=3
  out_port : Outport
  wires:
  bus_creator/1 -> out_port/1  "Subsystem2"
  EngVehicleSpThrottle2/1(out_port) -> bus_creator/1  "EngVehicleSpThrottle2"
  EngBrakeData/1(out_port) -> bus_creator/2  "EngBrakeData"
  EngVehicleSpThrottle/1(out_port) -> bus_creator/3  "EngVehicleSpThrottle"

== system P702_NI_SoftECU/Output/Subsystem2/To_NI_HIL/Soft_MRR ==
  MRR_Detection : Subsystem
  NumOfDetections : Constant  Value=0
  bus_creator : BusCreator  Inputs=2
  out_port : Outport
  wires:
  bus_creator/1 -> out_port/1  "Subsystem2"
  NumOfDetections/1 -> bus_creator/2  "NumOfDetections"
  MRR_Detection/1(out_port) -> bus_creator/1  "MRR_Detection"

== system P702_NI_SoftECU/Output/Subsystem2/To_NI_HIL/Soft_PCM ==
  EngBrakeData : Subsystem
  EngVehicleSpThottle2 : Subsystem
  EngVehicleSpThrottle : Subsystem
  EngineClimateData : Subsystem
  EngineClutchData : Subsystem
  EngineData_7 : Subsystem
  PowertrainData_10 : Subsystem
  TorqueDataEngFlags : Subsystem
  VehicleOperatingModes : Subsystem
  bus_creator : BusCreator  Inputs=9
  out_port : Outport
  wires:
  bus_creator/1 -> out_port/1  "Subsystem2"
  EngBrakeData/1(out_port) -> bus_creator/1  "EngBrakeData"
  EngineClimateData/1(out_port) -> bus_creator/2  "EngineClimateData"
  EngineClutchData/1(out_port) -> bus_creator/3  "EngineClutchData"
  EngVehicleSpThrottle/1(out_port) -> bus_creator/4  "EngVehicleSpThrottle"
  EngVehicleSpThottle2/1(out_port) -> bus_creator/5  "EngVehicleSpThottle2"
  VehicleOperatingModes/1(out_port) -> bus_creator/6  "VehicleOperatingModes"
  EngineData_7/1(out_port) -> bus_creator/7  "EngineData_7"
  TorqueDataEngFlags/1(out_port) -> bus_creator/8  "TorqueDataEngFlags"
  PowertrainData_10/1(out_port) -> bus_creator/9  "PowertrainData_10"

== system P702_NI_SoftECU/Output/Subsystem2/To_NI_HIL/Soft_PSCM ==
  Angle_SteeringWheel : Constant  Value=0
  StePinCompAnEst_D_Qf : Constant  Value=0
  StePinRelInit_An_Sns : Constant  Value=0
  StePw_B_Rq : Constant  Value=0
  SteWhlAngCounter : Constant  Value=0
  WhlAngleCs : Constant  Value=0
  bus_creator : BusCreator  Inputs=6
  out_port : Outport
  wires:
  bus_creator/1 -> out_port/1  "Subsystem2"
  Angle_SteeringWheel/1 -> bus_creator/1  "Angle_SteeringWheel"
  SteWhlAngCounter/1 -> bus_creator/2  "SteWhlAngCounter"
  WhlAngleCs/1 -> bus_creator/3  "WhlAngleCs"
  StePinRelInit_An_Sns/1 -> bus_creator/4  "StePinRelInit_An_Sns"
  StePw_B_Rq/1 -> bus_creator/5  "StePw_B_Rq"
  StePinCompAnEst_D_Qf/1 -> bus_creator/6  "StePinCompAnEst_D_Qf"

== system P702_NI_SoftECU/Output/Subsystem2/To_NI_HIL/Soft_RCM ==
  Accel_Data : Subsystem
  RCMStatusMessage2 : Subsystem
  Yaw_Data : Subsystem
  bus_creator : BusCreator  Inputs=3
  out_port : Outport
  wires:
  bus_creator/1 -> out_port/1  "Subsystem2"
  Accel_Data/1(out_port) -> bus_creator/1  "Accel_Data"
  Yaw_Data/1(out_port) -> bus_creator/2  "Yaw_Data"
  RCMStatusMessage2/1(out_port) -> bus_creator/3  "RCMStatusMessage2"

== system P702_NI_SoftECU/Output/Subsystem2/To_NI_HIL/Soft_SCCM ==
  Steering_Data : Subsystem
  Steering_Wheel_Data2 : Subsystem
  bus_creator : BusCreator  Inputs=2
  out_port : Outport
  wires:
  bus_creator/1 -> out_port/1  "Subsystem2"
  Steering_Data/1(out_port) -> bus_creator/1  "Steering_Data"
  Steering_Wheel_Data2/1(out_port) -> bus_creator/2  "Steering_Wheel_Data2"

== system P702_NI_SoftECU/Output/Subsystem2/To_NI_HIL/Soft_TCM ==
  TransGearData : Subsystem
  bus_creator : BusCreator  Inputs=1
  out_port : Outport
  wires:
  bus_creator/1 -> out_port/1  "Subsystem2"
  TransGearData/1(out_port) -> bus_creator/1  "TransGearData"

== system P702_NI_SoftECU/SoftECU/ABS/Logic/BrkDecel2MCPres ==
  note: Look up table from brake deceleration request to master cylinder pressure
  In1 : Inport
  Bus Creator : BusCreator  Inputs=1
  Bus Selector3 : BusSelector  OutputSignals=ADAS.ACCDATA_2.CmbbBrkDecel_A_Rq,ADAS.ACCDATA_2.CmbbBrkDecel_B_Rq
  Gain : Gain  Gain=-1
  LookUpTable : Lookup_n-D  NumberOfTableDimensions=1  BreakpointsForDimension1="[0   1  2   3   4     8     9     10     11     12     14]"  Table="[0   2 10  30 32   35   36    37     38    40     40 ]"  InternalRulePriority=Speed  RndMeth=Simplest  InputSameDT=on
  MinMax : MinMax  Function=max
  Mux : Mux  Inputs=2
  Product : Product
  Saturation : Saturate  UpperLimit=1  LowerLimit=0
  Transfer Fcn : TransferFcn  Denominator=[1 0.5]
  Out1 : Outport
  wires:
  In1/1 -> Bus Selector3/1
  Bus Selector3/1 -> Gain/1  "<CmbbBrkDecel_A_Rq>"
  Bus Selector3/2 -> Saturation/1  "<CmbbBrkDecel_B_Rq>"
  Saturation/1 -> Product/2
  Product/1 -> LookUpTable/1
  MinMax/1 -> Bus Creator/1  "MCPressure"
  Bus Creator/1 -> Out1/1  "ABSPhysical"
  Gain/1 -> Product/1
  Transfer Fcn/1 -> Mux/2
  Mux/1 -> MinMax/1
  LookUpTable/1 -> Mux/1, Transfer Fcn/1

== system P702_NI_SoftECU/SoftECU/ABS/Logic/BrkReqAcknowledges ==
  In1 : Inport
  Bus Selector3 : BusSelector  OutputSignals=ADAS.ACCDATA,ADAS.ACCDATA_2
  Bus Selector4 : BusSelector  OutputSignals=AccBrkPrchg_B_Rq,AccBrkDecel_B_Rq,AccStopStat_B_Rq,AccBrkTot_A_Rq
  Bus Selector5 : BusSelector  OutputSignals=CmbbBrkPrchg_D_Rq,CmbbBrkDecel_A_Rq,CmbbBaSens_D_Rq,CmbbBrkDecel_B_Rq
  Gain{,1..7} (8 alike) : Gain
  Terminator : Terminator
  Terminator1 : Terminator
  AccBrkPrchgActv_B_Actl : Outport
  AccBrkActv_B_Actl : Outport  Port=2
  AccStopActv_B_ActlBrk : Outport  Port=3
  CmbbBrkPrchg_B_Actl : Outport  Port=4
  CmbbBaSensInc_B_Actl : Outport  Port=5
  CmbbBrkDecel_B_Actl : Outport  Port=6
  wires:
  In1/1 -> Bus Selector3/1
  Bus Selector3/1 -> Bus Selector4/1  "<ACCDATA>"
  Bus Selector3/2 -> Bus Selector5/1  "<ACCDATA_2>"
  Bus Selector4/1 -> Gain/1  "<AccBrkPrchg_B_Rq>"
  Bus Selector4/2 -> Gain1/1  "<AccBrkDecel_B_Rq>"
  Bus Selector4/3 -> Gain2/1  "<AccStopStat_B_Rq>"
  Bus Selector4/4 -> Gain3/1  "<AccBrkTot_A_Rq>"
  Bus Selector5/1 -> Gain4/1  "<CmbbBrkPrchg_D_Rq>"
  Bus Selector5/2 -> Gain5/1  "<CmbbBrkDecel_A_Rq>"
  Bus Selector5/3 -> Gain6/1  "<CmbbBaSens_D_Rq>"
  Bus Selector5/4 -> Gain7/1  "<CmbbBrkDecel_B_Rq>"
  Gain3/1 -> Terminator/1
  Gain/1 -> AccBrkPrchgActv_B_Actl/1  "AccBrkPrchgActv_B_Actl"
  Gain1/1 -> AccBrkActv_B_Actl/1  "AccBrkActv_B_Actl"
  Gain2/1 -> AccStopActv_B_ActlBrk/1  "AccStopActv_B_ActlBrk"
  Gain4/1 -> CmbbBrkPrchg_B_Actl/1  "CmbbBrkPrchg_B_Actl"
  Gain5/1 -> Terminator1/1
  Gain6/1 -> CmbbBaSensInc_B_Actl/1  "CmbbBaSensInc_B_Actl"
  Gain7/1 -> CmbbBrkDecel_B_Actl/1  "CmbbBrkDecel_B_Actl"

== system P702_NI_SoftECU/SoftECU/ABS/Logic/Compute_VehVActlBrk_No_Cs ==
  Veh_V_ActlBrk : Inport
  VehVActlBrk_D_Qf : Inport  Port=2
  VehVActlBrk_No_Cnt : Inport  Port=3
  Bitwise Operator : simulink/Logic and Bit Operations/Bitwise Operator  logicop=AND  UseBitMask=on  BitMask=bin2dec('1111111100000000')  BitMaskRealWorld=Stored Integer
  Bitwise Operator1 : simulink/Logic and Bit Operations/Bitwise Operator  logicop=AND  UseBitMask=on  BitMask=bin2dec('0000000011111111')  BitMaskRealWorld=Stored Integer
  Bitwise Operator2 : simulink/Logic and Bit Operations/Bitwise Operator  logicop=NOT  UseBitMask=off  BitMask=bin2dec('11011001')  BitMaskRealWorld=Stored Integer
  Bitwise Operator3 : simulink/Logic and Bit Operations/Bitwise Operator  logicop=AND  UseBitMask=on  BitMask=bin2dec('0000000011111111')  BitMaskRealWorld=Stored Integer
  Bitwise Operator4 : simulink/Logic and Bit Operations/Bitwise Operator  logicop=AND  UseBitMask=on  BitMask=bin2dec('0000000011111111')  BitMaskRealWorld=Stored Integer
  Data Type Conversion{1..5,7} (6 alike) : DataTypeConversion  OutDataTypeStr=uint8
  Data Type Conversion6 : DataTypeConversion  OutDataTypeStr=uint16
  Scalling_factor : Gain  Gain=0.01
  Shift Arithmetic : ArithShift  BitShiftNumber=8
  Sum : Sum  Inputs=++++
  Terminator : Terminator
  VehVActlBrk_No_Cnt_In : simulink/Sources/Counter Limited  uplimit=15  tsamp=-1
  VehVActlBrk_No_Cs : Outport
  VehVActlBrk_No_Cnt1 : Outport  Port=2
  wires:
  Veh_V_ActlBrk/1 -> Scalling_factor/1
  Bitwise Operator/1 -> Shift Arithmetic/1
  Bitwise Operator3/1 -> Data Type Conversion2/1
  Bitwise Operator1/1 -> Data Type Conversion1/1
  Data Type Conversion1/1 -> Data Type Conversion3/1
  VehVActlBrk_D_Qf/1 -> Data Type Conversion7/1
  Sum/1 -> Bitwise Operator2/1
  Bitwise Operator2/1 -> VehVActlBrk_No_Cs/1  "VehVActlBrk_No_Cs"
  Data Type Conversion2/1 -> Sum/1  "Veh_V_ActlBrk_MSB"
  Data Type Conversion3/1 -> Sum/3  "VehVActlBrk_D_Qf"
  Data Type Conversion4/1 -> VehVActlBrk_No_Cnt1/1, Sum/4  "VehVActlBrk_No_Cnt"
  Data Type Conversion5/1 -> Sum/2  "Veh_V_ActlBrk_LSB"
  Bitwise Operator4/1 -> Data Type Conversion5/1
  Shift Arithmetic/1 -> Bitwise Operator3/1
  Data Type Conversion6/1 -> Bitwise Operator4/1, Bitwise Operator/1
  Data Type Conversion7/1 -> Bitwise Operator1/1
  Scalling_factor/1 -> Data Type Conversion6/1
  VehVActlBrk_No_Cnt_In/1 -> Data Type Conversion4/1  "VehVActlBrk_No_Cnt"
  VehVActlBrk_No_Cnt/1 -> Terminator/1

== system P702_NI_SoftECU/SoftECU/ABS/Logic/InvertYawRate ==
  note: JulianT:
      | TA Acces @ SingleProcessorModelTemplate/CPTIO_P1/SoftEcu/Input/Abs_PhyTA_CPTIO
  note: JulianT:
      | This subsystem is used to change the sign of yawrate in dependency on the connected camera ECU (IPMA)
      | 0: GENTEX
      | 1:DELPHI
  In1 : Inport
  IPMA_select_YawRate : Constant
  Switch_IPMA_Select : Switch  Criteria=u2 > Threshold
  invert1 : Gain  Gain=-1
  Out1 : Outport
  wires:
  In1/1 -> Switch_IPMA_Select/3, invert1/1
  invert1/1 -> Switch_IPMA_Select/1
  IPMA_select_YawRate/1 -> Switch_IPMA_Select/2
  Switch_IPMA_Select/1 -> Out1/1

== system P702_NI_SoftECU/SoftECU/ABS/Logic/VehicleStationary ==
  In1 : Inport
  Compare To Constant : simulink/Logic and Bit Operations/Compare To Constant  relop=<=  const=0.5  OutDataTypeStr=boolean
  dt_VehicleStationary : DataTypeConversion  RndMeth=Zero
  VehicleStationary : Outport
  wires:
  Compare To Constant/1 -> dt_VehicleStationary/1
  dt_VehicleStationary/1 -> VehicleStationary/1  "VehicleStationary"
  In1/1 -> Compare To Constant/1  "VehicleSpeed"
